simulink model "Examen_2_Sim"  (R2022a)
settings: Solver=VariableStepAuto  StartTime=0.0  StopTime=15  MaxStep=0.01  RelTol=1e-3
values from neighbouring files (symbols this model uses):
  A = [0 -1 3;-2 -4 -2;-4 3 -7]    [Examen_1_Script.m]    (also in Examen_2_Script.m)
  B = [-2;1;0]    [Examen_1_Script.m]    (also in Examen_2_Script.m)
  C = [8,4,5]    [Examen_1_Script.m]    (also in Examen_2_Script.m)
  K = lqr(A,B,Qc,Rc)    [Examen_2_Script.m]
  L2 = lqr(A',C',E*Sxi*E',Seta)'    [Examen_1_Script.m]    (also in Examen_2_Script.m; LQR.m = CLP)
  ue = Xe(4)    [Examen_1_Script.m]    (also in Examen_2_Script.m)
  x0 = [-5;-3;1]    [Examen_1_Script.m]    (also in Examen_2_Script.m)
  x0b = [0;0;0]    [Examen_1_Script.m]    (also in Examen_2_Script.m)
  xe = Xe(1:3)    [Examen_1_Script.m]    (also in Examen_2_Script.m)
  ye = 8    [Examen_1_Script.m]    (also in Examen_2_Script.m)
settings Model: Creator=fernando  LastModifiedBy=fernando

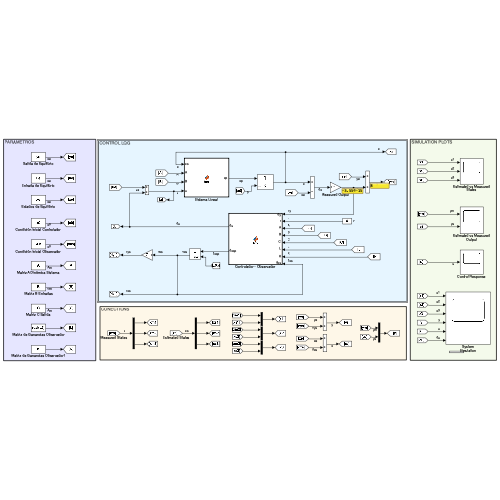
[thumbnail: Simulink's stored preview of the top-level diagram]
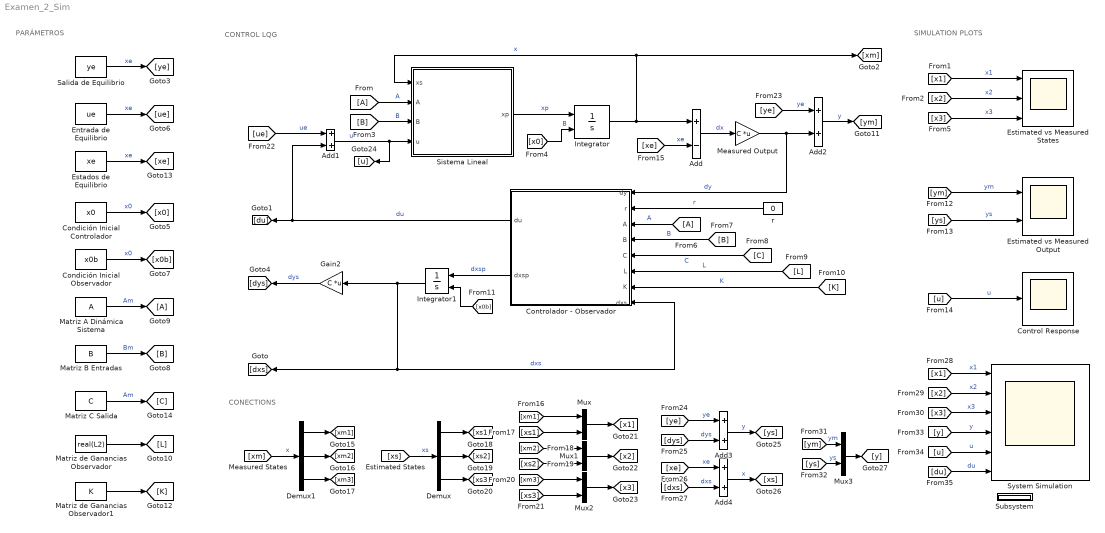
== system Examen_2_Sim ==
  note: CONECTIONS
  note: CONTROL LQG
  note: SIMULATION PLOTS
  note: PARÁMETROS
  " Matriz B Entradas" : Constant  Value=B  VectorParams1D=off
  " Matriz de Ganancias Observador" : Constant  Value=real(L2)  VectorParams1D=off
  " Matriz de Ganancias Observador1" : Constant  Value=K  VectorParams1D=off
  Add : Sum  Inputs=+-
  Add{1..4} (4 alike) : Sum
  Condición Inicial Controlador : Constant  Value=x0  VectorParams1D=off
  Condición Inicial Observador : Constant  Value=x0b  VectorParams1D=off
  Control Response : Scope
  Controlador - Observador : MATLAB Function  TreatAsAtomicUnit=on
  Demux : Demux  Outputs=3
  Demux1 : Demux  Outputs=3
  Entrada de Equilibrio : Constant  Value=ue  VectorParams1D=off
  Estados de Equilibrio : Constant  Value=xe  VectorParams1D=off
  Estimated vs Measured Output : Scope  NumInputPorts=2
  Estimated vs Measured States : Scope  NumInputPorts=3
  From : From
  From6 : From
  Gain2 : Gain  Gain=C  Multiplication=Matrix(K*u)
  Goto9 : Goto
  Integrator : Integrator  InitialConditionSource=external  InitialCondition=x0
  Integrator1 : Integrator  InitialConditionSource=external  InitialCondition=x0b
  Matriz A Dinámica Sistema : Constant  Value=A  VectorParams1D=off
  Matriz C Salida : Constant  Value=C  VectorParams1D=off
  Measured Output : Gain  Gain=C  Multiplication=Matrix(K*u)
  Mux{,1..3} (4 alike) : Mux  Inputs=2
  Salida de Equilibrio : Constant  Value=ye  VectorParams1D=off
  Sistema Lineal : MATLAB Function  TreatAsAtomicUnit=on
  Subsystem : Subsystem
  System Simulation : Scope  NumInputPorts=6
  r : Constant  Value=0  VectorParams1D=off
  wires:
  Salida de Equilibrio/1 -> [ye]  "xe"
  Condición Inicial Observador/1 -> [x0b]  "x0"
  " Matriz B Entradas"/1 -> [B]  "Bm"
  Matriz A Dinámica Sistema/1 -> Goto9/1  "Am"
  " Matriz de Ganancias Observador"/1 -> [L]
  " Matriz de Ganancias Observador1"/1 -> [K]
  Matriz C Salida/1 -> [C]  "Am"
  Condición Inicial Controlador/1 -> [x0]  "x0"
  Entrada de Equilibrio/1 -> [ue]  "xe"
  [C] -> Controlador - Observador/5(C)  "C"
  Sistema Lineal/1(xp) -> Integrator/1  "xp"
  From6/1 -> Controlador - Observador/3(A)  "A"
  r/1 -> Controlador - Observador/2(r)  "r"
  Controlador - Observador/2(dxsp) -> Integrator1/1  "dxsp"
  [L] -> Controlador - Observador/6(L)  "L"
  Gain2/1 -> [dys]  "dys"
  Integrator1/1 -> Gain2/1, Controlador - Observador/8(dxs), [dxs]  "dxs"
  Controlador - Observador/1(du) -> [du], Add1/2  "du"
  Measured Output/1 -> Controlador - Observador/1(dy), Add2/2  "dy"
  [B] -> Sistema Lineal/3(B)  "B"
  [B] -> Controlador - Observador/4(B)  "B"
  [K] -> Controlador - Observador/7(K)  "K"
  From/1 -> Sistema Lineal/2(A)  "A"
  [x0] -> Integrator/2  "B"
  [x0b] -> Integrator1/2
  Demux/1 -> [xs1]
  Demux/2 -> [xs2]
  Demux1/2 -> [xm2]
  Demux/3 -> [xs3]
  Demux1/3 -> [xm3]
  Demux1/1 -> [xm1]
  [xm] -> Demux1/1  "x"
  [xs] -> Demux/1  "xs"
  [xm1] -> Mux/1
  [xs1] -> Mux/2
  [xs2] -> Mux1/2
  [xm3] -> Mux2/1
  [xm2] -> Mux1/1
  [xs3] -> Mux2/2
  Mux2/1 -> [x3]
  Mux/1 -> [x1]
  Mux1/1 -> [x2]
  [x3] -> Estimated vs Measured States/3  "x3"
  [x2] -> Estimated vs Measured States/2  "x2"
  [x1] -> Estimated vs Measured States/1  "x1"
  [ym] -> Estimated vs Measured Output/1  "ym"
  [ys] -> Estimated vs Measured Output/2  "ys"
  [u] -> Control Response/1  "u"
  [xe] -> Add/2  "xe"
  Add/1 -> Measured Output/1  "dx"
  Integrator/1 -> Sistema Lineal/1(xs), [xm], Add/1  "x"
  Add1/1 -> [u], Sistema Lineal/4(u)  "u"
  [ue] -> Add1/1  "ue"
  Estados de Equilibrio/1 -> [xe]  "xe"
  Add2/1 -> [ym]  "y"
  [ye] -> Add2/1  "ye"
  [ye] -> Add3/1  "ye"
  Add3/1 -> [ys]  "y"
  [dys] -> Add3/2  "dys"
  [xe] -> Add4/1  "xe"
  Add4/1 -> [xs]  "x"
  [dxs] -> Add4/2  "dxs"
  [x2] -> System Simulation/2  "x2"
  [x1] -> System Simulation/1  "x1"
  [x3] -> System Simulation/3  "x3"
  [ym] -> Mux3/1  "ym"
  [ys] -> Mux3/2  "ys"
  Mux3/1 -> [y]
  [y] -> System Simulation/4  "y"
  [u] -> System Simulation/5  "u"
  [du] -> System Simulation/6  "du"

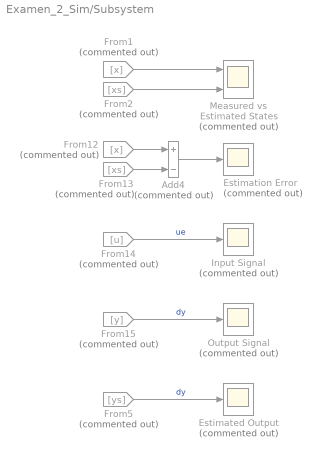
== system Examen_2_Sim/Subsystem ==
  Add4 : Sum  Commented=on  Inputs=+-
  Estimated Output : Scope  Commented=on
  Estimation Error : Scope  Commented=on
  From1 : From  Commented=on  GotoTag=x
  From12 : From  Commented=on  GotoTag=x
  From13 : From  Commented=on  GotoTag=xs
  From14 : From  Commented=on  GotoTag=u
  From15 : From  Commented=on  GotoTag=y
  From2 : From  Commented=on  GotoTag=xs
  From5 : From  Commented=on  GotoTag=ys
  Input Signal : Scope  Commented=on
  Measured vs Estimated States : Scope  Commented=on  NumInputPorts=2
  Output Signal : Scope  Commented=on
  wires:
  From5/1 -> Estimated Output/1  "dy"
  From13/1 -> Add4/2
  Add4/1 -> Estimation Error/1
  From15/1 -> Output Signal/1  "dy"
  From14/1 -> Input Signal/1  "ue"
  From12/1 -> Add4/1
  From1/1 -> Measured vs Estimated States/1
  From2/1 -> Measured vs Estimated States/2

== matlab function Examen_2_Sim/Sistema Lineal ==
  data: xs input; A input; B input; xp output; u input
function xp = fcn(xs,A,B,u)

xp = A*xs + B*u;

== matlab function Examen_2_Sim/Controlador - Observador ==
  data: dy input; r input; A input; B input; C input; L input; K input; du output; dxs input; dxsp output
function [du,dxsp] = fcn(dy,r,A,B,C,L,K,dxs)

dxsp = (A - L*C - B*K)*(dxs) + B*(r) + L*(dy);

du = -K*dxs + r;
